simulink model "switch_1"  (R2020a)
settings: Solver=VariableStepAuto  StartTime=0.0  StopTime=10.0  RelTol=1e-3
settings Model: Creator=Administrator  LastModifiedBy=Administrator

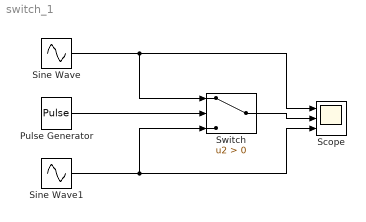
== system switch_1 ==
  Pulse Generator : DiscretePulseGenerator  PulseType=Time based  Period=1  PulseWidth=25
  Scope : Scope  NumInputPorts=3
  Sine Wave : Sin  SampleTime=0
  Sine Wave1 : Sin  Phase=-3.14  SampleTime=0
  Switch : Switch  Criteria=u2 > Threshold
  wires:
  Pulse Generator/1 -> Switch/2
  Sine Wave/1 -> Scope/1, Switch/1
  Sine Wave1/1 -> Scope/3, Switch/3
  Switch/1 -> Scope/2
